simulink model "Basic_Model_Open_Loop_softStart"  (R2025a)
settings: Solver=VariableStepAuto  StartTime=0.0  StopTime=150  RelTol=1e-3
libraries: spsControlledVoltageSourceLib x3, spsSeriesRLCBranchLib x3, spsVoltageMeasurementLib x3, spsCurrentMeasurementLib x1, spsDCMachineLib x1, spsDCVoltageSourceLib x1, spsDiodeLib x1, spsGroundLib x1, spsMosfetLib x1, spsPWMGeneratorDCDCLib x1, spsThreePhaseSourceLib x1, spsUniversalBridgeLib x1
settings Model: Creator=Josh  LastModifiedBy=kerim

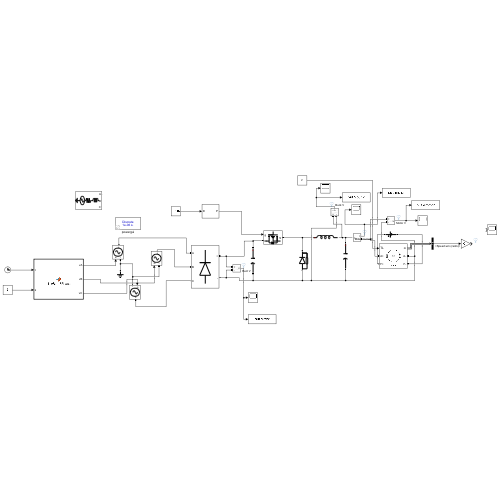
[thumbnail: Simulink's stored preview of the top-level diagram]
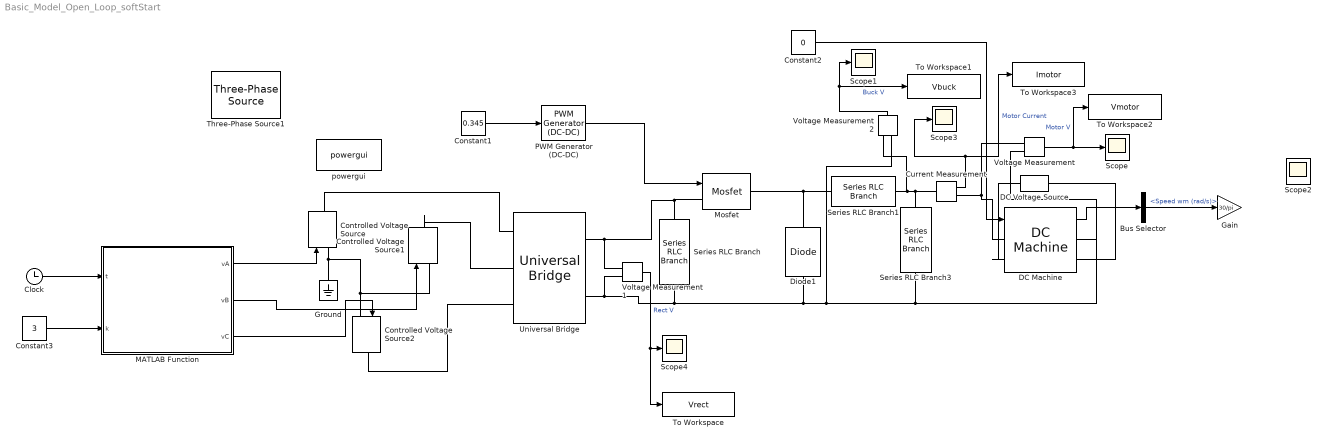
== system Basic_Model_Open_Loop_softStart ==
  Bus Selector : BusSelector  OutputSignals=Speed wm (rad/s)
  Clock : Clock
  Constant1 : Constant  Value=0.345
  Constant2 : Constant  Value=0
  Constant3 : Constant  Value=3
  Controlled Voltage Source : spsControlledVoltageSourceLib/Controlled Voltage Source  Initialize=on  Source_Type=AC  Amplitude=0  Phase=0  Frequency=0  Measurements=None
  Controlled Voltage Source1 : spsControlledVoltageSourceLib/Controlled Voltage Source  Initialize=on  Source_Type=AC  Amplitude=0  Phase=0  Frequency=0  Measurements=None
  Controlled Voltage Source2 : spsControlledVoltageSourceLib/Controlled Voltage Source  Initialize=on  Source_Type=AC  Amplitude=0  Phase=0  Frequency=0  Measurements=None
  Current Measurement : spsCurrentMeasurementLib/Current Measurement  PhasorSimulation=off  OutputType=Complex  PSBequivalent=0
  DC Machine : spsDCMachineLib/DC Machine  PresetModel=No  MechanicalLoad=Torque TL  FieldType=Wound  ShowDetailedParameters=on  MeasurementBus=off  RLa="[ 0.8  0.0125]"  RLf="[ 210  23]"  Laf=0.5  MachineConstant=Torque constant (N.m/A)  Ke=1.8  Kt=1.8  J=1  Bm=0  Tf=0  w0=0  Ifinit=1.04761904761905  TsPowergui=0  TsBlock=-1
  DC Voltage Source : spsDCVoltageSourceLib/DC Voltage Source  Amplitude=220  Measurements=None
  Diode1 : spsDiodeLib/Diode  Ron=0.001  Lon=0  Vf=0.8  IC=0  UseSnubber=0  Rs=500  Cs=250e-9  Measurements=off
  Gain : Gain  Gain=30/pi
  Ground : spsGroundLib/Ground  LConnTagsString=a
  MATLAB Function : MATLAB Function  TreatAsAtomicUnit=on
  Mosfet : spsMosfetLib/Mosfet  Ron=0.1  Lon=0  Rd=0.01  Vfd=0  IC=0  Rs=1e5  Cs=inf  Measurements=off
  PWM Generator (DC-DC) : spsPWMGeneratorDCDCLib/PWM Generator (DC-DC)  Fsw=50000  Ts=0
  Scope{,1..4} (5 alike) : Scope
      Scope settings: ActiveDisplayYMinimum=-195.14651777722787  ActiveDisplayYMaximum=323.369668767358  DataLoggingMaxPoints=200000000
      Scope1 settings: ActiveDisplayYMinimum=-1  ActiveDisplayYMaximum=1  DataLoggingMaxPoints=200000000
      Scope2 settings: ActiveDisplayYMinimum=-1  ActiveDisplayYMaximum=1  DataLoggingVariableName=ScopeData2
      Scope3 settings: ActiveDisplayYMinimum=-2.6221336428040489  ActiveDisplayYMaximum=8.7926283885998338  DataLoggingMaxPoints=200000000  DataLoggingVariableName=ScopeData3
      Scope4 settings: ActiveDisplayYMinimum=365.24041397079174  ActiveDisplayYMaximum=539.946102132254  DataLoggingMaxPoints=200000000  DataLoggingVariableName=ScopeData4
  Series RLC Branch : spsSeriesRLCBranchLib/Series RLC Branch  LConnTagsString=__new0  RConnTagsString=__new0  BranchType=C  Resistance=1  Inductance=1e-3  SetiL0=off  InitialCurrent=0  Capacitance=470e-6  Setx0=off  InitialVoltage=0  Measurements=None
  Series RLC Branch1 : spsSeriesRLCBranchLib/Series RLC Branch  LConnTagsString=__new0  RConnTagsString=__new0  BranchType=L  Resistance=1  Inductance=1.8e-3  SetiL0=off  InitialCurrent=0  Capacitance=1e-6  Setx0=off  InitialVoltage=0  Measurements=None
  Series RLC Branch3 : spsSeriesRLCBranchLib/Series RLC Branch  LConnTagsString=__new0  RConnTagsString=__new0  BranchType=C  Resistance=1  Inductance=1e-3  SetiL0=off  InitialCurrent=0  Capacitance=15e-6  Setx0=off  InitialVoltage=0  Measurements=None
  Three-Phase Source1 : spsThreePhaseSourceLib/Three-Phase Source  InternalConnection=Yg  VoltagePhases=off  Voltage=200*sqrt(2)  PhaseAngle=0  Voltage_phases=[25e3 25e3 25e3]/sqrt(3)  PhaseAngles_phases=[0 -120 +120]  Frequency=50  NonIdealSource=on  SpecifyImpedance=off  Resistance=0.001  Inductance=16.58e-9  ShortCircuitLevel=100e6  BaseVoltage=25e3  XRratio=7  BusType=swing  Pref=10e3  Qref=0  Prefabc=[10e3, 10e3, 10e3]  Qrefabc=[0, 0, 0]  Qmin=-inf  Qmax=inf
  To Workspace : ToWorkspace  VariableName=Vrect  SampleTime=-1
  To Workspace1 : ToWorkspace  VariableName=Vbuck  SampleTime=-1
  To Workspace2 : ToWorkspace  VariableName=Vmotor  SampleTime=-1
  To Workspace3 : ToWorkspace  VariableName=Imotor  SampleTime=-1
  Universal Bridge : spsUniversalBridgeLib/Universal Bridge  Arms=3  SnubberResistance=1e5  SnubberCapacitance=inf  Device=Diodes  Ron=1e-3  Lon=0  ForwardVoltages="[  0  0  ]"  ForwardVoltage=0  GTOparameters=[ 10e-6 , 20e-6 ]  IGBTparameters=[ 1e-6 , 2e-6 ]  Measurements=None  Measurements_2=None  converterType=Rectifier
  Voltage Measurement : spsVoltageMeasurementLib/Voltage Measurement  PhasorSimulation=off  OutputType=Complex  PSBequivalent=0
  Voltage Measurement1 : spsVoltageMeasurementLib/Voltage Measurement  PhasorSimulation=off  OutputType=Complex  PSBequivalent=0
  Voltage Measurement2 : spsVoltageMeasurementLib/Voltage Measurement  PhasorSimulation=off  OutputType=Complex  PSBequivalent=0
  powergui : sps_lib/powergui  Priority=1  SimulationMode=Discrete  SampleTime=1e-6  frequency=60  Iterations=50  frequencyindice=0  Pbase=100e6  ErrMax=1e-4  UnitsV=kV  UnitsW=MW  buscounter=0  FunctionMessages=off  echomessages=off  EnableUseOfTLC=off  CurrentSourceSwitches=off  DisableSnubberDevices=off  DisableRonSwitches=off  DisableVfSwitches=off  DisplayEquations=off  AutomaticDiscreteSolvers=off  SolverType=Tustin/Backward Euler (TBE)  Interpol=off  ExternalGateDelay=off  methode=off  Ts=100  x0status=blocks  SPID=on  SwTol=0  HookPort=off  NonlinearTolerance=1e-4  nMaxIteration=100  ContinueOnMaxIteration=off  RestoreLinks=warning  ResistiveCurrentMeasurement=off  Frange=[0:2:500]  Ylog=off  Xlog=on  ShowGrid=off  save=off  variable=ZData  structure=0  ZoomFFT=off  StartTime=0.0  cycles=1  DisplayStyle=1  fundamental=60  FreqAxis=off  MaxFrequency=1000  frequencyindicesteady=1  RmsSteady=1  display=off
  wires:
  PWM Generator (DC-DC)/1 -> Mosfet/1
  Voltage Measurement/1 -> To Workspace2/1, Scope/1  "Motor V"
  DC Machine/1 -> Bus Selector/1
  Bus Selector/1 -> Gain/1  "<Speed wm (rad/s)>"
  Current Measurement/1 -> Scope3/1, To Workspace3/1  "Motor Current"
  Constant1/1 -> PWM Generator (DC-DC)/1
  Voltage Measurement2/1 -> To Workspace1/1, Scope1/1  "Buck V"
  Clock/1 -> MATLAB Function/1(t)
  MATLAB Function/1(vA) -> Controlled Voltage Source/1
  MATLAB Function/2(vB) -> Controlled Voltage Source1/1
  MATLAB Function/3(vC) -> Controlled Voltage Source2/1
  Voltage Measurement1/1 -> To Workspace/1, Scope4/1  "Rect V"
  Constant2/1 -> DC Machine/1
  Constant3/1 -> MATLAB Function/2(k)
  connections:
  Series RLC Branch/LConn1 -- Mosfet/LConn1 -- Voltage Measurement1/LConn1 -- Universal Bridge/RConn1
  Universal Bridge/RConn2 -- Voltage Measurement1/LConn2 -- Voltage Measurement/LConn2 -- DC Machine/RConn1 -- Series RLC Branch3/RConn1 -- Voltage Measurement2/LConn2 -- Diode1/LConn1 -- Series RLC Branch/RConn1
  Diode1/RConn1 -- Series RLC Branch1/LConn1 -- Mosfet/RConn1
  Series RLC Branch1/RConn1 -- Voltage Measurement2/LConn1 -- Current Measurement/LConn1 -- Series RLC Branch3/LConn1
  DC Machine/LConn2 -- DC Voltage Source/RConn1
  DC Machine/RConn2 -- DC Voltage Source/LConn1
  Voltage Measurement/LConn1 -- DC Machine/LConn1 -- Current Measurement/RConn1
  Controlled Voltage Source/LConn1 -- Ground/LConn1 -- Controlled Voltage Source2/LConn1 -- Controlled Voltage Source1/LConn1
  Controlled Voltage Source2/RConn1 -- Universal Bridge/LConn3
  Controlled Voltage Source1/RConn1 -- Universal Bridge/LConn2
  Controlled Voltage Source/RConn1 -- Universal Bridge/LConn1

== matlab function Basic_Model_Open_Loop_softStart/MATLAB Function ==
  data: t input; vA output; vB output; vC output; k input
function [vA, vB, vC] = slowStart3Phase(t, k)
    vA = min(t*k,200*sqrt(2))*sin(2*pi*50*t);
    vB = min(t*k,200*sqrt(2))*sin(2*pi*50*t - 2*pi/3);
    vC = min(t*k,200*sqrt(2))*sin(2*pi*50*t - 4*pi/3);
end
